simulink model "tethersNCsContrl_th"  (R2018b)
settings: Solver=VariableStepAuto  StartTime=0.0  StopTime=1  RelTol=1e-3
values from neighbouring files (symbols this model uses):
  alti_sp = 10    [tethersNCsContrl_ts.m]
  euler = [0;0;0]*pi/180    [tethersNCsContrl_ts.m]
  flow = [0;0;0]    [tethersNCsContrl_ts.m]
  OwB = [0;0;0]    [tethersNCsContrl_ts.m]
  pitch_sp = 1*pi/180    (= 0.0174532925199)    [tethersNCsContrl_ts.m]
  Rcm_o = zeros(3,1)    [tethersNCsContrl_ts.m]
  roll_sp = 1*pi/180    (= 0.0174532925199)    [tethersNCsContrl_ts.m]
  Vcm_o = zeros(3,1)    [tethersNCsContrl_ts.m]
libraries: tethersNCsContrl_cl x1
settings Model: Creator=Ayaz  LastModifiedBy=Ayaz

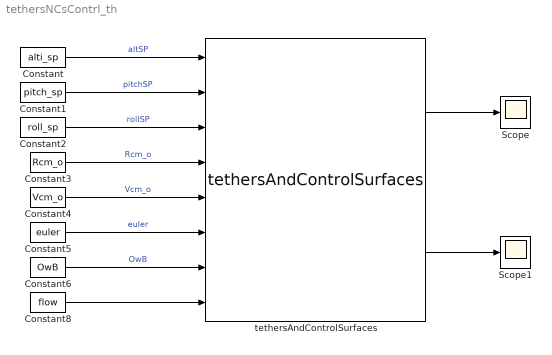
== system tethersNCsContrl_th ==
  Constant : Constant  Value=alti_sp  VectorParams1D=off
  Constant1 : Constant  Value=pitch_sp  VectorParams1D=off
  Constant2 : Constant  Value=roll_sp  VectorParams1D=off
  Constant3 : Constant  Value=Rcm_o  VectorParams1D=off
  Constant4 : Constant  Value=Vcm_o  VectorParams1D=off
  Constant5 : Constant  Value=euler  VectorParams1D=off
  Constant6 : Constant  Value=OwB  VectorParams1D=off
  Constant8 : Constant  Value=flow  VectorParams1D=off
  Scope : Scope
  Scope1 : Scope
  tethersAndControlSurfaces : tethersNCsContrl_cl/tethersAndControlSurfaces  thr_clr=ctrllr.tethers  cs_clr=ctrllr.controlSurfaces
  wires:
  Constant/1 -> tethersAndControlSurfaces/1  "altSP"
  Constant1/1 -> tethersAndControlSurfaces/2  "pitchSP"
  Constant2/1 -> tethersAndControlSurfaces/3  "rollSP"
  Constant3/1 -> tethersAndControlSurfaces/4  "Rcm_o"
  Constant4/1 -> tethersAndControlSurfaces/5  "Vcm_o"
  Constant5/1 -> tethersAndControlSurfaces/6  "euler"
  Constant6/1 -> tethersAndControlSurfaces/7  "OwB"
  Constant8/1 -> tethersAndControlSurfaces/8
  tethersAndControlSurfaces/1 -> Scope/1
  tethersAndControlSurfaces/2 -> Scope1/1
